simulink model "lab6dsim"  (R2022b)
settings: Solver=FixedStepAuto  StartTime=0.0  StopTime=1.9*10.0  FixedStep=10/(1024*32)  RelTol=1e-3
undefined symbols (not defined in the file or in its folder): DiscIntNeverNeededParam, lutdata, lutix
libraries: dsparch4 x2
settings Model: Creator=andjog  LastModifiedBy=andjog

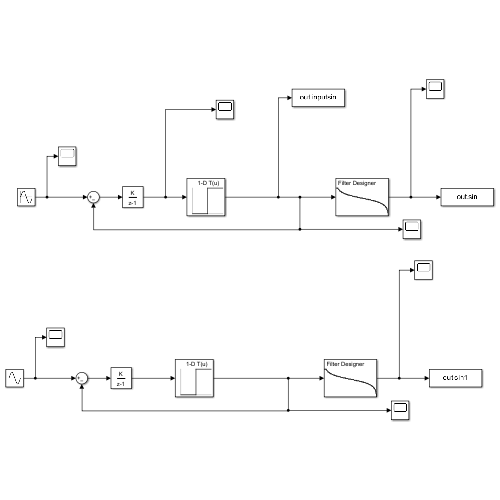
[thumbnail: Simulink's stored preview of the top-level diagram]
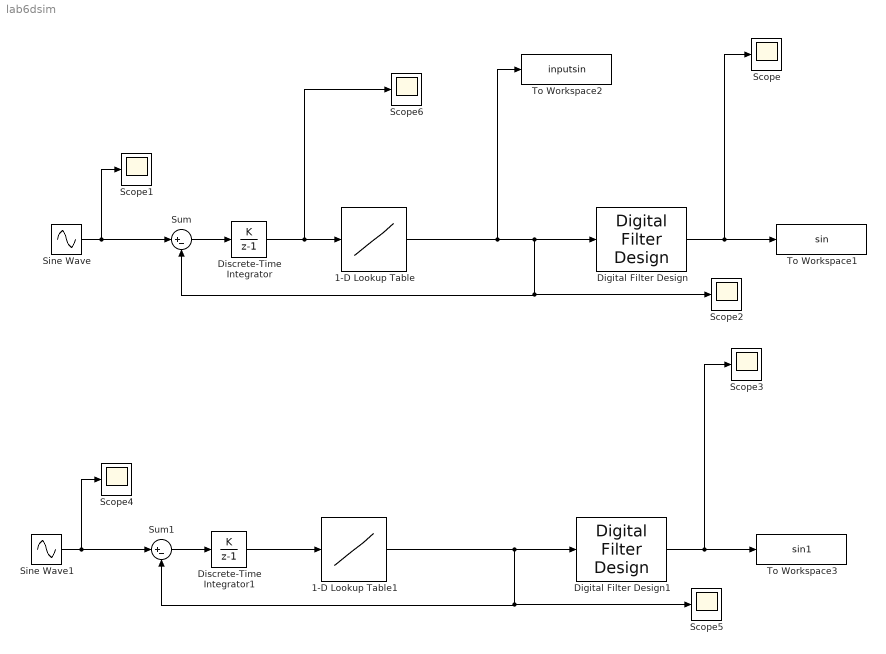
== system lab6dsim ==
  1-D Lookup Table : Lookup_n-D  NumberOfTableDimensions=1  BreakpointsForDimension1=lutix(2)  Table=lutdata(2)  InternalRulePriority=Speed  RndMeth=Simplest
  1-D Lookup Table1 : Lookup_n-D  NumberOfTableDimensions=1  BreakpointsForDimension1=lutix(2)  Table=lutdata(2)  InternalRulePriority=Speed  RndMeth=Simplest
  Digital Filter Design : dsparch4/Digital Filter Design  mwdsp_browser_bugfix_var=off
  Digital Filter Design1 : dsparch4/Digital Filter Design  mwdsp_browser_bugfix_var=off
  Discrete-Time Integrator : DiscreteIntegrator  IntegratorMethod=Accumulation: Forward Euler  SampleTime=-1  ICPrevOutput=DiscIntNeverNeededParam  ICPrevScaledInput=DiscIntNeverNeededParam
  Discrete-Time Integrator1 : DiscreteIntegrator  IntegratorMethod=Accumulation: Forward Euler  SampleTime=-1  ICPrevOutput=DiscIntNeverNeededParam  ICPrevScaledInput=DiscIntNeverNeededParam
  Scope{,1..6} (7 alike) : Scope
  Sine Wave : Sin  Amplitude=0  Bias=0.01  Frequency=pi  SampleTime=0
  Sine Wave1 : Sin  Amplitude=0  Bias=0.001  Frequency=pi  SampleTime=0
  Sum : Sum  Inputs=|+-
  Sum1 : Sum  Inputs=|+-
  To Workspace1 : ToWorkspace  VariableName=sin  SaveFormat=Structure With Time  SampleTime=-1
  To Workspace2 : ToWorkspace  VariableName=inputsin  SaveFormat=Structure With Time  SampleTime=-1
  To Workspace3 : ToWorkspace  VariableName=sin1  SaveFormat=Structure With Time  SampleTime=-1
  wires:
  Sum/1 -> Discrete-Time Integrator/1
  Discrete-Time Integrator/1 -> Scope6/1, 1-D Lookup Table/1
  1-D Lookup Table/1 -> Digital Filter Design/1, Scope2/1, Sum/2, To Workspace2/1
  Sine Wave/1 -> Scope1/1, Sum/1
  Digital Filter Design/1 -> Scope/1, To Workspace1/1
  Discrete-Time Integrator1/1 -> 1-D Lookup Table1/1
  Sum1/1 -> Discrete-Time Integrator1/1
  Digital Filter Design1/1 -> Scope3/1, To Workspace3/1
  Sine Wave1/1 -> Scope4/1, Sum1/1
  1-D Lookup Table1/1 -> Digital Filter Design1/1, Scope5/1, Sum1/2
